simulink model "LP_TP_realData"  (R2013a)
settings: Solver=ode45  StartTime=0.0  StopTime=100.0  RelTol=1e-3
libraries: dsparch4 x3, visionanalysis x1, dspsrcs4 x1
settings Model: Creator=cg  LastModifiedBy=cg

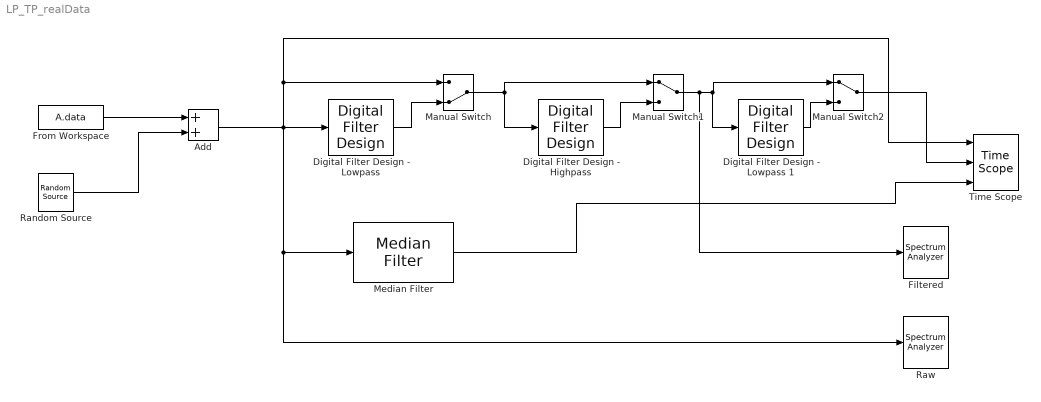
== system LP_TP_realData ==
  Add : Sum
  "Digital Filter Design - Lowpass " : dsparch4/Digital Filter Design  mwdsp_browser_bugfix_var=off
  Digital Filter Design - Lowpass 1 : dsparch4/Digital Filter Design  mwdsp_browser_bugfix_var=off
  "Digital Filter Design - Highpass " : dsparch4/Digital Filter Design  mwdsp_browser_bugfix_var=off
  Filtered : SpectrumAnalyzer
      settings: CopyFcn=scopeextensions.ScopeBlock.callback(gcbh, 'onBlockCopy', gcbh);  DeleteFcn=scopeextensions.ScopeBlock.callback(gcbh, 'onBlockDelete');  PreSaveFcn=scopeextensions.ScopeBlock.callback(gcbh, 'onModelSave');  NameChangeFcn=scopeextensions.ScopeBlock.callback(gcbh, 'onBlockRename');  CloseFcn=scopeextensions.ScopeBlock.callback(gcbh, 'onBlockClose');  PreDeleteFcn=scopeextensions.ScopeBlock.callback(gcbh, 'onBlockPreDelete');
  From Workspace : FromWorkspace  VariableName=A.data  OutDataTypeStr=double  SampleTime=1/1000
  Manual Switch : ManualSwitch  CurrentSetting=0
  Manual Switch1 : ManualSwitch
  Manual Switch2 : ManualSwitch
  Median Filter : visionanalysis/Median Filter  nghbood=[26 1]  outSize=Same as input port I  padType=Constant  padSrc=Specify via dialog  padVal=0  roundingMode=Floor  overflowMode=off
  Random Source : dspsrcs4/Random Source  SrcType=Uniform  NormMethod=Ziggurat  CltLength=12  MinVal=0  MaxVal=1  MeanVal=0  VarVal=1  RepMode=Not repeatable  rawSeed=1  IsInherit=off  SampMode=Discrete  SampTime=1/1000  SampFrame=4095  DataType=Double  OutComplex=Real
  Raw : SpectrumAnalyzer
      settings: CopyFcn=scopeextensions.ScopeBlock.callback(gcbh, 'onBlockCopy', gcbh);  DeleteFcn=scopeextensions.ScopeBlock.callback(gcbh, 'onBlockDelete');  PreSaveFcn=scopeextensions.ScopeBlock.callback(gcbh, 'onModelSave');  NameChangeFcn=scopeextensions.ScopeBlock.callback(gcbh, 'onBlockRename');  CloseFcn=scopeextensions.ScopeBlock.callback(gcbh, 'onBlockClose');  PreDeleteFcn=scopeextensions.ScopeBlock.callback(gcbh, 'onBlockPreDelete');
  Time Scope : TimeScope  NumInputPorts=3  DefaultConfigurationName=spbscopes.TimeScopeBlockCfg
      settings: CopyFcn=scopeextensions.ScopeBlock.callback(gcbh, 'onBlockCopy', gcbh);  DeleteFcn=scopeextensions.ScopeBlock.callback(gcbh, 'onBlockDelete');  PreSaveFcn=scopeextensions.ScopeBlock.callback(gcbh, 'onModelSave');  NameChangeFcn=scopeextensions.ScopeBlock.callback(gcbh, 'onBlockRename');  OpenFcn=scopeextensions.SrcWiredSL.coreBlockCommand('Open',gcbh)  CloseFcn=scopeextensions.ScopeBlock.callback(gcbh, 'onBlockClose');  PreDeleteFcn=scopeextensions.ScopeBlock.callback(gcbh, 'onBlockPreDelete');
  wires:
  Manual Switch/1 -> "Digital Filter Design - Highpass "/1, Manual Switch1/1
  Manual Switch1/1 -> Digital Filter Design - Lowpass 1/1, Manual Switch2/1, Filtered/1
  Manual Switch2/1 -> Time Scope/2
  Digital Filter Design - Lowpass 1/1 -> Manual Switch2/2
  Add/1 -> Median Filter/1, Raw/1, Time Scope/1, Manual Switch/1, "Digital Filter Design - Lowpass "/1
  "Digital Filter Design - Highpass "/1 -> Manual Switch1/2
  "Digital Filter Design - Lowpass "/1 -> Manual Switch/2
  Median Filter/1 -> Time Scope/3
  From Workspace/1 -> Add/1
  Random Source/1 -> Add/2
